simulink model "Part1DesignKF_2017b"  (R2017b)
settings: Solver=ode45  StartTime=0.0  StopTime=200  FixedStep=Ts  RelTol=1e-3  EnableMultiTasking=on
values from neighbouring files (symbols this model uses):
  alfa1 = .2    (= 0.2)    [parameters.m]
  alfa2 = .2    (= 0.2)    [parameters.m]
  b1 = 0.1    [init_kalman.m]    (also in kalm.m; parameters.m)
  b2 = 0.1    [init_kalman.m]    (also in kalm.m; parameters.m)
  b3_nom = 0.1    [parameters.m]
  b4_nom = 0.1    [parameters.m]
  b5 = 0.1    [init_kalman.m]    (also in kalm.m; parameters.m)
  k1 = 0.15    [init_kalman.m]    (also in kalm.m; parameters.m)
  k3_nom = .1    (= 0.1)    [parameters.m]
  k4_nom = .1    (= 0.1)    [parameters.m]
  m1 = 1    [parameters.m]
  m2 = 1    [parameters.m]
  m3 = 1    [parameters.m]
  m4 = 1    [parameters.m]
  Ts = 0.001    [init_kalman.m]    (also in kalm.m; parameters.m)
undefined symbols (not defined in the file or in its folder): A_D_Re_GNARC, B_D_Re_GNARC, C_D_Re_GNARC, D_D_Re_GNARC
libraries: simulink x4
settings Model: Creator=VAHiD  LastModifiedBy=Toni
settings DataIOCC: LimitDataPoints=on  SaveFormat=Array
settings OptimizationCC: ExpressionDepthLimit=2147483647  LifeSpan=inf
settings DebuggingCC: UnderspecifiedInitializationDetection=Classic  MergeDetectMultiDrivingBlocksExec=none  SolverPrmCheckMsg=warning  FcnCallInpInsideContextMsg=warning  StateNameClashWarn=warning  SFUnexpectedBacktrackingDiag=warning  SFNoUnconditionalDefaultTransitionDiag=warning  SFExecutionAtInitializationDiag=none
settings HardwareCC: ProdBitPerPointer=32  ProdBitPerSizeT=32  ProdBitPerPtrDiffT=32  ProdLargestAtomicFloat=None  ProdIntDivRoundTo=Undefined  ProdEndianess=Unspecified  ProdWordSize=32  ProdHWDeviceType=32-bit Generic
settings ModelReferenceCC: PropagateSignalLabelsOutOfModel=off
settings CodeAppCC: StateflowObjectComments=on
settings GRTTargetCC: TargetLangStandard=C89/C90 (ANSI)  GeneratePreprocessorConditionals=Disable all  CombineOutputUpdateFcns=off  GRTInterface=on
settings ConfigComp: CovMetricSettings=dw  CovHtmlReporting=on  CovSaveCumulativeToWorkspaceVar=on  CovSaveSingleToWorkspaceVar=on  CovExternalEMLEnable=off

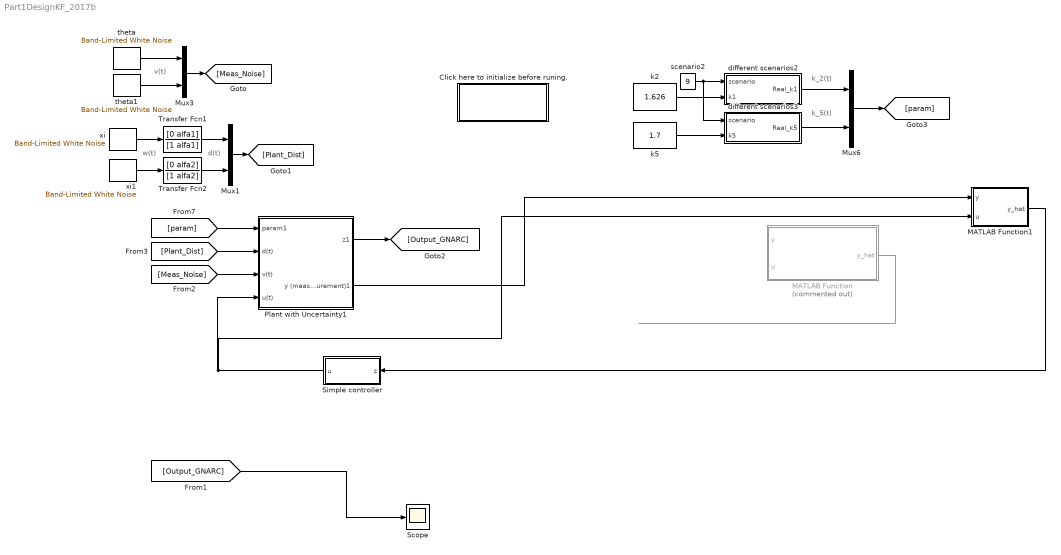
== system Part1DesignKF_2017b ==
  note: w(t)
  note: v(t)
  note: d(t)
  note: k_2(t)
  note: k_5(t)
  Click here to initialize before runing. : Subsystem
      settings: OpenFcn=start_up
      mask Display: disp('Load\Parameters')
  MATLAB Function : MATLAB Function  Commented=on  TreatAsAtomicUnit=on
  MATLAB Function1 : MATLAB Function  TreatAsAtomicUnit=on
  Mux1 : Mux  Inputs=2
  Mux3 : Mux  Inputs=2
  Mux6 : Mux  Inputs=2
  Plant with Uncertainty1 : Subsystem
  Scope : Scope
  Simple controller : Subsystem
  Transfer Fcn1 : TransferFcn  Numerator=[0 alfa1]  Denominator=[1 alfa1]
  Transfer Fcn2 : TransferFcn  Numerator=[0 alfa2]  Denominator=[1 alfa2]
  different scenarios2 : Subsystem
  different scenarios3 : Subsystem
  k2 : Constant  Value=1.626
  k5 : Constant  Value=1.7
  scenario2 : Constant  Value=9
  theta : simulink/Sources/Band-Limited White Noise  Cov=TH1  Ts=Ts  seed=1
  theta1 : simulink/Sources/Band-Limited White Noise  Cov=TH2  Ts=Ts  seed=2
  xi : simulink/Sources/Band-Limited White Noise  Cov=XI1  Ts=Ts  seed=3
  xi1 : simulink/Sources/Band-Limited White Noise  Cov=XI2  Ts=Ts  seed=4
  wires:
  Mux3/1 -> [Meas_Noise]
  theta/1 -> Mux3/1
  theta1/1 -> Mux3/2
  Mux1/1 -> [Plant_Dist]
  xi/1 -> Transfer Fcn1/1
  xi1/1 -> Transfer Fcn2/1
  Transfer Fcn1/1 -> Mux1/1
  Transfer Fcn2/1 -> Mux1/2
  scenario2/1 -> different scenarios2/1(scenario), different scenarios3/1(scenario)
  k2/1 -> different scenarios2/2(k1)
  k5/1 -> different scenarios3/2(k5)
  different scenarios3/1(Real_k5) -> Mux6/2
  different scenarios2/1(Real_k1) -> Mux6/1
  Mux6/1 -> [param]
  [param] -> Plant with Uncertainty1/1(param1)
  [Plant_Dist] -> Plant with Uncertainty1/2(d(t))
  [Meas_Noise] -> Plant with Uncertainty1/3(v(t))
  Plant with Uncertainty1/1(z1) -> [Output_GNARC]
  Plant with Uncertainty1/2(y (measurement)1) -> MATLAB Function1/1(y)
  Simple controller/1(u) -> MATLAB Function1/2(u), Plant with Uncertainty1/4(u(t))
  [Output_GNARC] -> Scope/1
  MATLAB Function1/1(y_hat) -> Simple controller/1(z)
  MATLAB Function/1(y_hat) -> ?

== system Part1DesignKF_2017b/Click here to initialize before runing. ==

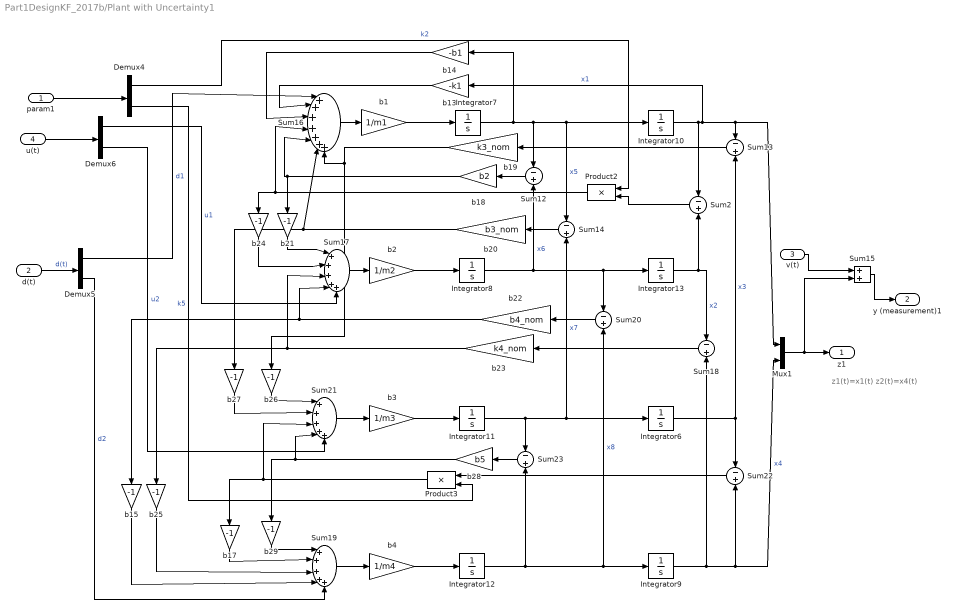
== system Part1DesignKF_2017b/Plant with Uncertainty1 ==
  note: z1(t)=x1(t)
      | z2(t)=x4(t)
  param1 : Inport
  d(t) : Inport  Port=2
  v(t) : Inport  Port=3
  u(t) : Inport  Port=4
  Demux4 : Demux  Outputs=2
  Demux5 : Demux  Outputs=2
  Demux6 : Demux  Outputs=2
  Integrator{6..13} (8 alike) : Integrator
  Mux1 : Mux  Inputs=2
  Product2 : Product  SaturateOnIntegerOverflow=on  InputSameDT=on  OutDataTypeStr=Inherit: Same as first input
  Product3 : Product  SaturateOnIntegerOverflow=on  InputSameDT=on  OutDataTypeStr=Inherit: Same as first input
  Sum{2,12..14,18,20,22..23} (8 alike) : Sum  Inputs=-+  SaturateOnIntegerOverflow=on  InputSameDT=on  OutDataTypeStr=Inherit: Same as first input
  Sum15 : Sum  SaturateOnIntegerOverflow=on  InputSameDT=on  OutDataTypeStr=Inherit: Same as first input
  Sum16 : Sum  Inputs=|+++++++  SaturateOnIntegerOverflow=on  InputSameDT=on  OutDataTypeStr=Inherit: Same as first input
  Sum17 : Sum  Inputs=|+++++  SaturateOnIntegerOverflow=on  InputSameDT=on  OutDataTypeStr=Inherit: Same as first input
  Sum19 : Sum  Inputs=|+++++  SaturateOnIntegerOverflow=on  InputSameDT=on  OutDataTypeStr=Inherit: Same as first input
  Sum21 : Sum  Inputs=|+++++  SaturateOnIntegerOverflow=on  InputSameDT=on  OutDataTypeStr=Inherit: Same as first input
  b1 : Gain  Gain=1/m1  SaturateOnIntegerOverflow=on  OutDataTypeStr=Inherit: Same as input  ParamDataTypeStr=Inherit: Same as input
  b13 : Gain  Gain=-k1  SaturateOnIntegerOverflow=on  OutDataTypeStr=Inherit: Same as input  ParamDataTypeStr=Inherit: Same as input
  b14 : Gain  Gain=-b1  SaturateOnIntegerOverflow=on  OutDataTypeStr=Inherit: Same as input  ParamDataTypeStr=Inherit: Same as input
  b{15,17,21,24..27,29} (8 alike) : Gain  Gain=-1  SaturateOnIntegerOverflow=on  OutDataTypeStr=Inherit: Same as input  ParamDataTypeStr=Inherit: Same as input
  b18 : Gain  Gain=b2  SaturateOnIntegerOverflow=on  OutDataTypeStr=Inherit: Same as input  ParamDataTypeStr=Inherit: Same as input
  b19 : Gain  Gain=k3_nom  SaturateOnIntegerOverflow=on  OutDataTypeStr=Inherit: Same as input  ParamDataTypeStr=Inherit: Same as input
  b2 : Gain  Gain=1/m2  SaturateOnIntegerOverflow=on  OutDataTypeStr=Inherit: Same as input  ParamDataTypeStr=Inherit: Same as input
  b20 : Gain  Gain=b3_nom  SaturateOnIntegerOverflow=on  OutDataTypeStr=Inherit: Same as input  ParamDataTypeStr=Inherit: Same as input
  b22 : Gain  Gain=b4_nom  SaturateOnIntegerOverflow=on  OutDataTypeStr=Inherit: Same as input  ParamDataTypeStr=Inherit: Same as input
  b23 : Gain  Gain=k4_nom  SaturateOnIntegerOverflow=on  OutDataTypeStr=Inherit: Same as input  ParamDataTypeStr=Inherit: Same as input
  b28 : Gain  Gain=b5  SaturateOnIntegerOverflow=on  OutDataTypeStr=Inherit: Same as input  ParamDataTypeStr=Inherit: Same as input
  b3 : Gain  Gain=1/m3  SaturateOnIntegerOverflow=on  OutDataTypeStr=Inherit: Same as input  ParamDataTypeStr=Inherit: Same as input
  b4 : Gain  Gain=1/m4  SaturateOnIntegerOverflow=on  OutDataTypeStr=Inherit: Same as input  ParamDataTypeStr=Inherit: Same as input
  z1 : Outport
  y (measurement)1 : Outport  Port=2
  wires:
  Sum15/1 -> y (measurement)1/1
  v(t)/1 -> Sum15/1
  param1/1 -> Demux4/1
  Mux1/1 -> Sum15/2, z1/1
  d(t)/1 -> Demux5/1  "d(t)"
  u(t)/1 -> Demux6/1
  b25/1 -> Sum19/3
  b15/1 -> Sum19/4
  Demux5/2 -> Sum19/5  "d2"
  Integrator7/1 -> b14/1, Sum12/1, Integrator10/1, Sum14/1  "x5"
  Integrator10/1 -> b13/1, Sum13/1, Mux1/1, Sum2/1  "x1"
  Integrator8/1 -> Sum12/2, Integrator13/1, Sum20/1  "x6"
  Integrator11/1 -> Integrator6/1, Sum14/2, Sum23/1  "x7"
  Integrator12/1 -> Integrator9/1, Sum20/2, Sum23/2  "x8"
  Demux5/1 -> Sum16/1  "d1"
  b13/1 -> Sum16/2
  b14/1 -> Sum16/3
  Integrator13/1 -> Sum2/2, Sum18/1  "x2"
  Sum2/1 -> Product2/2
  Demux4/1 -> Product2/1  "k2"
  Sum12/1 -> b18/1
  b18/1 -> Sum16/5, b21/1
  Integrator6/1 -> Sum13/2, Sum22/1  "x3"
  Sum13/1 -> b19/1
  Sum14/1 -> b20/1
  b20/1 -> Sum16/6, b27/1
  Sum16/1 -> b1/1
  Product2/1 -> Sum16/4, b24/1
  Integrator9/1 -> Sum18/2, Sum22/2, Mux1/2  "x4"
  Sum18/1 -> b23/1
  b23/1 -> Sum17/3, b25/1
  Sum17/1 -> b2/1
  Sum20/1 -> b22/1
  b22/1 -> Sum17/4, b15/1
  b21/1 -> Sum17/1
  b24/1 -> Sum17/2
  Demux6/1 -> Sum17/5  "u1"
  Sum21/1 -> b3/1
  b19/1 -> Sum16/7, b26/1
  b26/1 -> Sum21/1
  b27/1 -> Sum21/2
  Sum22/1 -> Product3/1
  Product3/1 -> Sum21/3, b17/1
  Demux4/2 -> Product3/2  "k5"
  Sum23/1 -> b28/1
  b28/1 -> Sum21/4, b29/1
  Demux6/2 -> Sum21/5  "u2"
  Sum19/1 -> b4/1
  b17/1 -> Sum19/2
  b29/1 -> Sum19/1
  b1/1 -> Integrator7/1
  b2/1 -> Integrator8/1
  b3/1 -> Integrator11/1
  b4/1 -> Integrator12/1

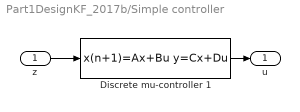
== system Part1DesignKF_2017b/Simple controller ==
  z : Inport
  Discrete mu-controller 1 : DiscreteStateSpace  Description=disp('sss')  A=A_D_Re_GNARC  B=B_D_Re_GNARC  C=C_D_Re_GNARC  D=D_D_Re_GNARC  SampleTime=Ts
  u : Outport
  wires:
  z/1 -> Discrete mu-controller 1/1
  Discrete mu-controller 1/1 -> u/1

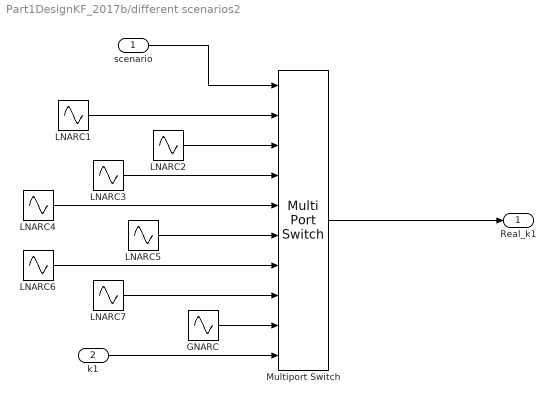
== system Part1DesignKF_2017b/different scenarios2 ==
  scenario : Inport
  k1 : Inport  Port=2
  GNARC : Sin  Amplitude=.75  Bias=1  Frequency=2*pi/700  Phase=-pi/2  SampleTime=0
  LNARC1 : Sin  Amplitude=.875  Bias=1.625  Frequency=2*pi/700  Phase=-pi/2  SampleTime=0
  LNARC2 : Sin  Amplitude=.55/2  Bias=.775  Frequency=2*pi/700  Phase=-pi/2  SampleTime=0
  LNARC3 : Sin  Amplitude=.75/2  Bias=1.4250  Frequency=2*pi/700  Phase=-pi/2  SampleTime=0
  LNARC4 : Sin  Amplitude=.15/2  Bias=.325  Frequency=2*pi/700  Phase=-pi/2  SampleTime=0
  LNARC5 : Sin  Amplitude=.15  Bias=.55  Frequency=2*pi/700  Phase=-pi/2  SampleTime=0
  LNARC6 : Sin  Amplitude=.45/2  Bias=.925  Frequency=2*pi/700  Phase=-pi/2  SampleTime=0
  LNARC7 : Sin  Amplitude=.30  Bias=1.45  Frequency=2*pi/700  Phase=-pi/2  SampleTime=0
  Multiport Switch : MultiPortSwitch  Inputs=9
  Real_k1 : Outport
  wires:
  Multiport Switch/1 -> Real_k1/1
  scenario/1 -> Multiport Switch/1
  LNARC3/1 -> Multiport Switch/4
  LNARC6/1 -> Multiport Switch/7
  LNARC7/1 -> Multiport Switch/8
  LNARC5/1 -> Multiport Switch/6
  LNARC4/1 -> Multiport Switch/5
  LNARC1/1 -> Multiport Switch/2
  LNARC2/1 -> Multiport Switch/3
  k1/1 -> Multiport Switch/10
  GNARC/1 -> Multiport Switch/9

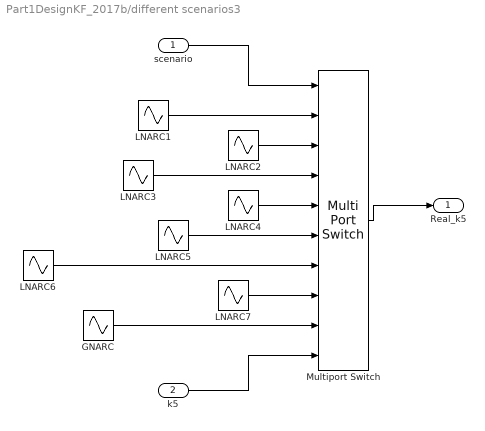
== system Part1DesignKF_2017b/different scenarios3 ==
  scenario : Inport
  k5 : Inport  Port=2
  GNARC : Sin  Amplitude=1.6  Bias=1.8  Frequency=2*pi/700  Phase=-pi/2  SampleTime=0
  LNARC1 : Sin  Amplitude=.8  Bias=1.7  Frequency=2*pi/700  Phase=-3*pi/2  SampleTime=0
  LNARC2 : Sin  Amplitude=.8  Bias=2.6  Frequency=2*pi/700  Phase=-pi/2  SampleTime=0
  LNARC3 : Sin  Amplitude=.8  Bias=2.6  Frequency=2*pi/700  Phase=-pi/2  SampleTime=0
  LNARC{4..7} (4 alike) : Sin  Amplitude=.8  Bias=1  Frequency=2*pi/700  Phase=-pi/2  SampleTime=0
  Multiport Switch : MultiPortSwitch  Inputs=9
  Real_k5 : Outport
  wires:
  LNARC5/1 -> Multiport Switch/6
  LNARC7/1 -> Multiport Switch/8
  LNARC6/1 -> Multiport Switch/7
  LNARC3/1 -> Multiport Switch/4
  scenario/1 -> Multiport Switch/1
  Multiport Switch/1 -> Real_k5/1
  k5/1 -> Multiport Switch/10
  GNARC/1 -> Multiport Switch/9
  LNARC1/1 -> Multiport Switch/2
  LNARC2/1 -> Multiport Switch/3
  LNARC4/1 -> Multiport Switch/5

== matlab function Part1DesignKF_2017b/MATLAB Function1 ==
  settings: updateMethod=DISCRETE
  data: y input; u input; y_hat output
function y_hat  = kalm2(y,u)
% this function is a Kalman filter that
% returns the estimate y_hat based on the noisy measurement and control u
% 

persistent x_hat
if isempty(x_hat)
    x_hat = zeros(10,1);
end

PHI =     [1.0000    0.0000    0.0000    0.0000    0.0010    0.0000    0.0000    0.0000    0.0000    0.0000
    0.0000    1.0000    0.0000    0.0000    0.0000    0.0010    0.0000    0.0000    0.0000    0.0000
    0.0000    0.0000    1.0000    0.0000    0.0000    0.0000    0.0010    0.0000    0.0000    0.0000
    0.0000    0.0000    0.0000    1.0000    0.0000    0.0000    0.0000    0.0010    0.0000    0.0000
   -0.0019    0.0016    0.0001    0.0000    0.9997    0.0001    0.0001    0.0000    0.0010    0.0000
    0.0016   -0.0017    0.0000    0.0001    0.0001    0.9998    0.0000    0.0001    0.0000    0.0000
    0.0001    0.0000    0.0016    0.0017    0.0001    0.0000    0.9998    0.0001    0.0000    0.0000
    0.0000    0.0001    0.0017   -0.0018    0.0000    0.0001    0.0001    0.9998    0.0000    0.0010
         0         0         0         0         0         0         0         0    0.9998         0
         0         0         0         0         0         0         0         0         0    0.9998];

DELTA = 1.0e-03*[ 0.0000    0.0000
    0.0005    0.0000
    0.0000    0.0005
    0.0000    0.0000
    0.0001    0.0001
    0.9999    0.0000
    0.0000    0.9999
    0.0001    0.0001
         0         0
         0         0];

GAMMA = 1.0e-03* [0.0000    0.0000
    0.0000    0.0000
    0.0000    0.0000
    0.0000    0.0000
    0.0001    0.0000
    0.0000    0.0000
    0.0000    0.0000
    0.0000    0.0001
    0.2000         0
         0    0.2000];

C = zeros(2,10);
C(1,1)=1;
C(2,4)=1;

K = [    0.0110    0.0003   
         0.0001    0.0001
         0.0328    0.2739
         0.0003    0.0135
         0.0605    0.0034
         0.0028    0.0015
         0.0395    0.3231
         0.0034    0.0911
         0.1814   -0.0374
        -0.0371   -0.1135];

x_hat = PHI*x_hat + DELTA*u + K*(y-C*x_hat);

x = x_hat;
y_hat = C*x_hat;

end

== matlab function Part1DesignKF_2017b/MATLAB Function ==
  settings: updateMethod=DISCRETE
  data: y input; u input; y_hat output
function y_hat  = kalm(y,u)

J_M1 = 1;
J_M2 = 1;
J_L1 = 1;
J_L2 = 1;
k1 = 0.15;
k2 = 1.625;
k3 = 0.1;
k4 = 0.1;
k5 = 1.7;
Ts = 0.001;
b1 = 0.1; b2 = 0.1; b3 = 0.1; b4 =0.1; b5 = 0.1;

persistent P_
if isempty(P_)
    P_ = zeros(10,10);
end

A = [zeros(4,4) eye(4) zeros(4,2);
    -(k1+k2+k1)/J_L1 k2/J_L1 k3/J_L1 0 -(b1+b2+b3)/J_L1 b2/J_L1 b3/J_L1 0 1/J_L1 0;
    k2/J_M1 -(k2+k4)/J_M1 0 k4/J_M1 b2/J_M1 -(b2+b4)/J_M1 0 b4/J_M1 0 0;
    k3/J_M2 0 (-k3+k5)/J_M2 k5/J_M2 b3/J_M2 0 -(b3+b5)/J_M2 b5/J_M2 0 0;
    0 k4/J_L2 k5/J_L2 -(k4+k5)/J_L2 0 b4/J_L2 b5/J_L2 -(b4+b5)/J_L2 0 1/J_L2;
    0 0 0 0 0 0 0 0 -0.2 0;
    0 0 0 0 0 0 0 0 0 -0.2];
B = zeros(10,2);
B(6,1)=1/J_M1;
B(7,2)=1/J_M1;
G = zeros(10,2);
G(9,1)=0.2;
G(10,2)=0.2;
C = zeros(2,10);
C(1,1)=1;
C(2,4)=1;

% noise covariance matrices
Q = 1*eye(2);       % unity intensity on process noise
R = 10^-6*eye(2);   % 10^-6 intensity on measurement noise
    
%sys = ss(A,[B G], C, 0);

%[kest, L, P, M, Z] = kalmd(sys, Q, R, Ts);

persistent x
if isempty(x)
    x = zeros(10,1);
end


PHI =     [1.0000    0.0000    0.0000    0.0000    0.0010    0.0000    0.0000    0.0000    0.0000    0.0000
    0.0000    1.0000    0.0000    0.0000    0.0000    0.0010    0.0000    0.0000    0.0000    0.0000
    0.0000    0.0000    1.0000    0.0000    0.0000    0.0000    0.0010    0.0000    0.0000    0.0000
    0.0000    0.0000    0.0000    1.0000    0.0000    0.0000    0.0000    0.0010    0.0000    0.0000
   -0.0019    0.0016    0.0001    0.0000    0.9997    0.0001    0.0001    0.0000    0.0010    0.0000
    0.0016   -0.0017    0.0000    0.0001    0.0001    0.9998    0.0000    0.0001    0.0000    0.0000
    0.0001    0.0000    0.0016    0.0017    0.0001    0.0000    0.9998    0.0001    0.0000    0.0000
    0.0000    0.0001    0.0017   -0.0018    0.0000    0.0001    0.0001    0.9998    0.0000    0.0010
         0         0         0         0         0         0         0         0    0.9998         0
         0         0         0         0         0         0         0         0         0    0.9998];

DELTA = 1.0e-03*[ 0.0000    0.0000
    0.0005    0.0000
    0.0000    0.0005
    0.0000    0.0000
    0.0001    0.0001
    0.9999    0.0000
    0.0000    0.9999
    0.0001    0.0001
         0         0
         0         0];

GAMMA = 1.0e-03* [0.0000    0.0000
    0.0000    0.0000
    0.0000    0.0000
    0.0000    0.0000
    0.0001    0.0000
    0.0000    0.0000
    0.0000    0.0000
    0.0000    0.0001
    0.2000         0
         0    0.2000];

K = P_*transpose(C)*inv(C*P_*transpose(C)+R);
x_hat = x + K*(y-C*x);
P_hat = (eye(10)-K*C)*P_*transpose(eye(10)-K*C)+K*R*transpose(K);

x = PHI*x_hat+DELTA*u;
P_ = PHI*P_hat*transpose(PHI)+GAMMA*Q*transpose(GAMMA);

x_hat = x;
y_hat = C*x;

end
